simulink model "fft_test"  (Simulink 7.0)
settings: Solver=VariableStepDiscrete  StartTime=0.0  StopTime=500  RelTol=1e-3
undefined symbols (not defined in the file or in its folder): bit_rev
libraries: xbsIndex_r4 x960, casper_library x89
(part 1 of 10)
settings Model: Creator=User  LastModifiedBy=User
settings DebuggingCC: SaveWithDisabledLinksMsg=none  SaveWithParameterizedLinksMsg=none

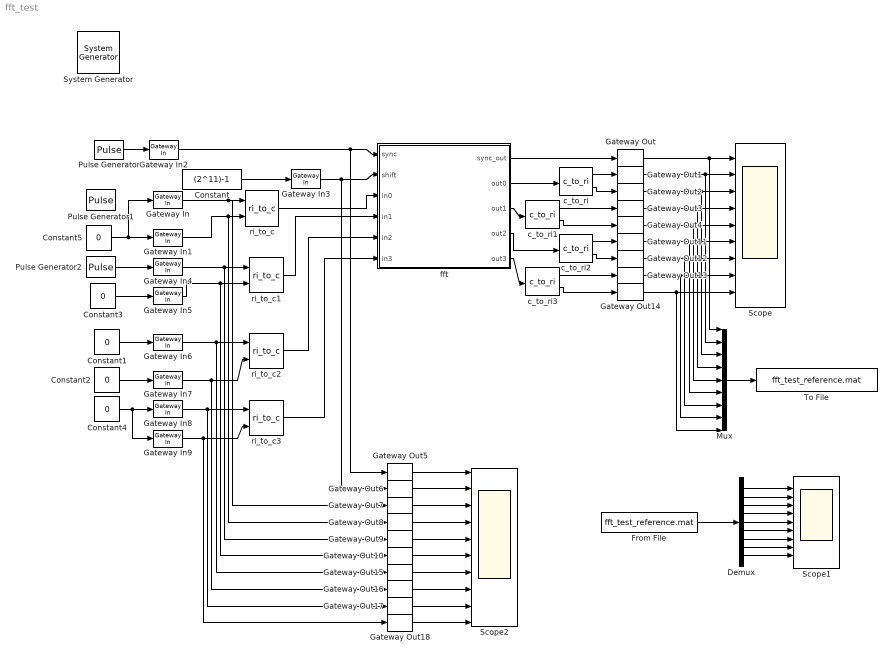
== system fft_test ==
  " System Generator" : xbsIndex_r4/ System Generator  Tag=genX  SystemSampleTime=-1  xilinxfamily=Virtex4  part=xc4vsx35  speed=-10  package=ff668  synthesis_tool=XST  clock_wrapper=Clock Enables  directory=./netlist  testbench=off  simulink_period=1  sysclk_period=100  dcm_input_clock_period=100  incr_netlist=off  trim_vbits=Everywhere in SubSystem  dbl_ovrd=According to Block Masks  core_generation=According to Block Masks  run_coregen=off  deprecated_control=off  eval_field=0  block_type=sysgen
      settings: block_version=10.1.1
  Constant : Constant  Value=(2^11)-1  OutDataType=sfix(16)  OutScaling=2^0
  Constant{1..5} (5 alike) : Constant  Value=0  OutDataType=sfix(16)  OutScaling=2^0
  Demux : Demux  Outputs=9
  From File : FromFile  FileName=fft_test_reference.mat  SampleTime=1
  Gateway In{,1,4..9} (8 alike) : xbsIndex_r4/Gateway In  arith_type="Signed  (2's comp)"  n_bits=8  bin_pt=7  quantization=Truncate  overflow=Wrap  period=1  dbl_ovrd=off  timing_constraint=None  locs_specified=off  LOCs={}  block_type=gatewayin
      settings: infoedit="Gateway in block.  Converts inputs of type Simulink integer, double and fixed point to  Xilinx fixed point type.<P><P>Hardware notes:  In hardware these blocks become top level input ports."  block_version=10.1.1
  Gateway In2 : xbsIndex_r4/Gateway In  arith_type=Boolean  n_bits=18  bin_pt=17  quantization=Truncate  overflow=Wrap  period=1  dbl_ovrd=off  timing_constraint=None  locs_specified=off  LOCs={}  block_type=gatewayin
      settings: infoedit="Gateway in block.  Converts inputs of type Simulink integer, double and fixed point to  Xilinx fixed point type.<P><P>Hardware notes:  In hardware these blocks become top level input ports."  block_version=10.1.1
  Gateway In3 : xbsIndex_r4/Gateway In  arith_type=Unsigned  n_bits=11  bin_pt=0  quantization=Truncate  overflow=Wrap  period=1  dbl_ovrd=off  timing_constraint=None  locs_specified=off  LOCs={}  block_type=gatewayin
      settings: infoedit="Gateway in block.  Converts inputs of type Simulink integer, double and fixed point to  Xilinx fixed point type.<P><P>Hardware notes:  In hardware these blocks become top level input ports."  block_version=10.1.1
  Gateway Out{,1..18} (19 alike) : xbsIndex_r4/Gateway Out  hdl_port=on  timing_constraint=None  locs_specified=off  LOCs={}  block_type=gatewayout
      settings: infoedit="Gateway out block.  Converts Xilinx fixed point inputs into ouputs of type Simulink integer, double, or fixed point.<P><P>Hardware notes:  In hardware these blocks become top level output ports or are discarded, depending on how they are configured."  block_version=10.1.1
  Mux : Mux  Inputs=9
  Pulse Generator : DiscretePulseGenerator  Period=2^7  PhaseDelay=11
  Pulse Generator1 : DiscretePulseGenerator  Amplitude=0.5  Period=2^4  PhaseDelay=12
  Pulse Generator2 : DiscretePulseGenerator  Amplitude=0.5  Period=2^5  PhaseDelay=12
  Scope : Scope  NumInputPorts=9
      settings: YMin=-1~0~0~-5~-5~-5~-5~-5~-5  YMax=2~1~1~5~5~5~5~5~5
  Scope1 : Scope  NumInputPorts=9
      settings: YMin=-1~0~0~-5~-5~-5~-5~-5~-5  YMax=2~1~1~5~5~5~5~5~5
  Scope2 : Scope  NumInputPorts=10
      settings: YMin=-1~0~0~-5~-5~-5~-5~-5~-5~-5  YMax=2~1~1~5~5~5~5~5~5~5  SaveName=ScopeData2
  To File : ToFile  Filename=fft_test_reference.mat  MatrixName=reference
  c_to_ri{,1..3} (4 alike) : casper_library/Misc/c_to_ri  SystemSampleTime=-1  n_bits=8  bin_pt=7
      settings: AttributesFormatString=8_7 r/i
  fft : Subsystem  AncestorBlock=casper_library/FFTs/fft  mask(fft){FFTSize=6, BitWidth=8, n_inputs=2, quantization=Round  (unbiased: +/- Inf), overflow=Saturate, add_latency=2, mult_latency=3, bram_latency=1}
      mask prompts: FFTSize "Size of FFT: (2^?)"; BitWidth "Bit Width"; n_inputs "Number of Simultaneous Inputs: (2^?)"; quantization "Quantization Behavior"; overflow "Overflow Behavior"; add_latency "Add Latency"; mult_latency "Mult Latency"; bram_latency "BRAM Latency"
      mask init:
      | fft_init(gcb,...
      |     'FFTSize', FFTSize,...
      |     'BitWidth', BitWidth,...
      |     'n_inputs', n_inputs,...
      |     'quantization', quantization,...
      |     'overflow', overflow,...
      |     'add_latency', add_latency,...
      |     'mult_latency', mult_latency,...
      |     'bram_latency', bram_latency);
      settings: AttributesFormatString=FFTSize=6, n_inputs=2
      mask StyleString: edit,edit,edit,popup(Truncate|Round  (unbiased: +/- Inf)|Round  (unbiased: Even Values)),popup(Wrap|Saturate|Error),edit,edit,edit
  ri_to_c{,1..3} (4 alike) : casper_library/Misc/ri_to_c  SystemSampleTime=-1
  wires:
  Pulse Generator/1 -> Gateway In2/1
  Gateway In2/1 -> fft/1(sync), Gateway Out5/1
  Constant/1 -> Gateway In3/1
  Gateway In3/1 -> fft/2(shift), Gateway Out6/1
  fft/1(sync_out) -> Gateway Out/1
  fft/2(out0) -> c_to_ri/1
  c_to_ri/1 -> Gateway Out1/1
  c_to_ri/2 -> Gateway Out2/1
  c_to_ri1/2 -> Gateway Out4/1
  fft/3(out1) -> c_to_ri1/1
  c_to_ri1/1 -> Gateway Out3/1
  Gateway Out/1 -> Scope/1, Mux/1
  Gateway In/1 -> ri_to_c/1, Gateway Out7/1
  Gateway In1/1 -> ri_to_c/2, Gateway Out8/1
  Gateway In4/1 -> ri_to_c1/1, Gateway Out9/1
  Gateway In5/1 -> ri_to_c1/2, Gateway Out10/1
  Gateway Out1/1 -> Scope/2, Mux/2
  Gateway Out2/1 -> Scope/3, Mux/3
  Mux/1 -> To File/1
  Demux/1 -> Scope1/1
  Demux/2 -> Scope1/2
  Demux/3 -> Scope1/3
  Demux/4 -> Scope1/4
  Demux/5 -> Scope1/5
  Gateway Out5/1 -> Scope2/1
  Gateway Out6/1 -> Scope2/2
  Gateway Out7/1 -> Scope2/3
  Gateway Out8/1 -> Scope2/4
  Gateway Out9/1 -> Scope2/5
  Gateway Out10/1 -> Scope2/6
  Constant2/1 -> Gateway In7/1
  Constant4/1 -> Gateway In8/1, Gateway In9/1
  Gateway In6/1 -> ri_to_c2/1, Gateway Out15/1
  Gateway In7/1 -> ri_to_c2/2, Gateway Out16/1
  Gateway In8/1 -> ri_to_c3/1, Gateway Out17/1
  Gateway In9/1 -> ri_to_c3/2, Gateway Out18/1
  ri_to_c/1 -> fft/3(in0)
  ri_to_c1/1 -> fft/4(in1)
  ri_to_c2/1 -> fft/5(in2)
  ri_to_c3/1 -> fft/6(in3)
  fft/4(out2) -> c_to_ri2/1
  fft/5(out3) -> c_to_ri3/1
  c_to_ri2/1 -> Gateway Out11/1
  c_to_ri2/2 -> Gateway Out12/1
  c_to_ri3/1 -> Gateway Out13/1
  c_to_ri3/2 -> Gateway Out14/1
  Gateway Out3/1 -> Scope/4, Mux/4
  Gateway Out4/1 -> Scope/5, Mux/5
  Gateway Out11/1 -> Scope/6, Mux/6
  Gateway Out12/1 -> Scope/7, Mux/7
  Gateway Out13/1 -> Scope/8, Mux/8
  Gateway Out14/1 -> Scope/9, Mux/9
  Gateway Out15/1 -> Scope2/7
  Gateway Out16/1 -> Scope2/8
  Gateway Out17/1 -> Scope2/9
  Gateway Out18/1 -> Scope2/10
  From File/1 -> Demux/1
  Demux/6 -> Scope1/6
  Demux/7 -> Scope1/7
  Demux/8 -> Scope1/8
  Demux/9 -> Scope1/9
  Constant3/1 -> Gateway In5/1
  Constant1/1 -> Gateway In6/1
  Pulse Generator2/1 -> Gateway In4/1
  Constant5/1 -> Gateway In1/1, Gateway In/1

== system fft_test/fft ==
  sync : Inport  OutDataType=sfix(16)  OutScaling=2^0
  shift : Inport  Port=2  OutDataType=sfix(16)  OutScaling=2^0
  in0 : Inport  Port=3
  in1 : Inport  Port=4
  in2 : Inport  Port=5
  in3 : Inport  Port=6
  fft_biplex0 : Subsystem  AncestorBlock=casper_library/FFTs/fft_biplex  mask(fft_biplex){FFTSize=4, BitWidth=8, quantization=Round  (unbiased: +/- Inf), overflow=Saturate, add_latency=2, mult_latency=3, bram_latency=1}
      mask prompts: FFTSize "Size of FFT: (2^? pnts)"; BitWidth "Bitwidth: (Max Efficiency at 18 bits)"; quantization "Quantization Behavior"; overflow "Overflow Behavior"; add_latency "Add Latency"; mult_latency "Mult Latency"; bram_latency "BRAM Latency"
      mask init:
      | fft_biplex_init(gcb,...
      |     'FFTSize', FFTSize,...
      |     'BitWidth', BitWidth,...
      |     'quantization', quantization,...
      |     'overflow', overflow,...
      |     'add_latency', add_latency,...
      |     'mult_latency', mult_latency,...
      |     'bram_latency', bram_latency);
      settings: AttributesFormatString=FFTSize=4, BitWidth=8
      mask StyleString: edit,edit,popup(Truncate|Round  (unbiased: +/- Inf)|Round  (unbiased: Even Values)),popup(Wrap|Saturate|Error),edit,edit,edit
  fft_biplex1 : Subsystem  AncestorBlock=casper_library/FFTs/fft_biplex  mask(fft_biplex){FFTSize=4, BitWidth=8, quantization=Round  (unbiased: +/- Inf), overflow=Saturate, add_latency=2, mult_latency=3, bram_latency=1}
      mask prompts: FFTSize "Size of FFT: (2^? pnts)"; BitWidth "Bitwidth: (Max Efficiency at 18 bits)"; quantization "Quantization Behavior"; overflow "Overflow Behavior"; add_latency "Add Latency"; mult_latency "Mult Latency"; bram_latency "BRAM Latency"
      mask init: same as fft_test/fft/fft_biplex0
      settings: AttributesFormatString=FFTSize=4, BitWidth=8
      mask StyleString: edit,edit,popup(Truncate|Round  (unbiased: +/- Inf)|Round  (unbiased: Even Values)),popup(Wrap|Saturate|Error),edit,edit,edit
  fft_direct : Subsystem  AncestorBlock=casper_library/FFTs/fft_direct  mask(fft_direct){FFTSize=2, BitWidth=8, add_latency=2, mult_latency=3, bram_latency=1, quantization=Round  (unbiased: +/- Inf), overflow=Saturate, MapTail=1, LargerFFTSize=6, StartStage=5}
      mask prompts: FFTSize "Size of FFT: (2^?)"; BitWidth "Bit Width"; add_latency "Add Latency"; mult_latency "Mult Latency"; bram_latency "BRAM Latency"; quantization "Quantization Behavior"; overflow "Overflow Behavior"; MapTail "Map Tail of Larger FFT"; LargerFFTSize "Size of Larger FFT (2^?):"; StartStage "Start Stage of Map Tail:"
      mask help:
      | Implements an N-point FFT with the classic
      | butterfly structure with N inputs and N outputs
      mask init:
      | fft_direct_init(gcb,...
      |     'FFTSize', FFTSize,...
      |     'BitWidth', BitWidth,...
      |     'add_latency', add_latency,...
      |     'mult_latency', mult_latency,...
      |     'bram_latency', bram_latency,...
      |     'quantization', quantization,...
      |     'overflow', overflow,...
      |     'MapTail', MapTail,...
      |     'LargerFFTSize', LargerFFTSize,...
      |     'StartStage', StartStage);
      settings: AttributesFormatString=FFTSize=2
      mask StyleString: edit,edit,edit,edit,edit,popup(Truncate|Round  (unbiased: +/- Inf)|Round  (unbiased: Even Values)),popup(Wrap|Saturate|Error),edit,edit,edit
  fft_unscrambler : Subsystem  AncestorBlock=casper_library/FFTs/fft_unscrambler  mask(fft_unscrambler){FFTSize=6, n_inputs=2, bram_latency=1}
      mask prompts: FFTSize "Size of FFT: (2^?)"; n_inputs "Number of Simultaneous Inputs: (2^?)"; bram_latency "BRAM Latency"
      mask init:
      | fft_unscrambler_init(gcb,...
      |     'FFTSize',FFTSize,... 
      |     'n_inputs', n_inputs,...
      |     'bram_latency', bram_latency);
      settings: AttributesFormatString=FFTSize=6, n_inputs=2
  slice : xbsIndex_r4/Slice  nbits=2  boolean_output=off  mode=Lower Bit Location + Width  bit1=0  base1=MSB of Input  bit0=4  base0=LSB of Input  dbl_ovrd=off  block_type=slice
      settings: infoedit="Extracts a given range of bits from each input sample and presents it at the output.  The output type is ordinarily unsigned with binary point at zero, but can be Boolean when the slice is one bit wide.<P><P>Hardware notes: In hardware this block costs nothing."  block_version=10.1.1
  sync_out : Outport  OutDataType=sfix(16)  OutScaling=2^0
  out0 : Outport  Port=2  OutDataType=sfix(16)  OutScaling=2^0
  out1 : Outport  Port=3  OutDataType=sfix(16)  OutScaling=2^0
  out2 : Outport  Port=4
  out3 : Outport  Port=5
  wires:
  in0/1 -> fft_biplex0/1(pol1)
  in1/1 -> fft_biplex0/2(pol2)
  shift/1 -> fft_biplex0/4(shift), fft_biplex1/4(shift), slice/1
  sync/1 -> fft_biplex0/3(sync), fft_biplex1/3(sync)
  in2/1 -> fft_biplex1/1(pol1)
  in3/1 -> fft_biplex1/2(pol2)
  slice/1 -> fft_direct/2(shift)
  fft_biplex0/4(sync_out) -> fft_direct/1(sync)
  fft_biplex0/1(pol1_out) -> fft_direct/3(in0)
  fft_biplex0/2(pol2_out) -> fft_direct/4(in1)
  fft_biplex1/1(pol1_out) -> fft_direct/5(in2)
  fft_biplex1/2(pol2_out) -> fft_direct/6(in3)
  fft_direct/1(sync_out) -> fft_unscrambler/1(sync)
  fft_unscrambler/1(sync_out) -> sync_out/1
  fft_direct/2(out0) -> fft_unscrambler/2(In1)
  fft_unscrambler/2(Out1) -> out0/1
  fft_direct/3(out1) -> fft_unscrambler/3(In2)
  fft_unscrambler/3(Out2) -> out1/1
  fft_direct/4(out2) -> fft_unscrambler/4(In3)
  fft_unscrambler/4(Out3) -> out2/1
  fft_direct/5(out3) -> fft_unscrambler/5(In4)
  fft_unscrambler/5(Out4) -> out3/1

== system fft_test/fft/fft_biplex0 ==
  pol1 : Inport  OutDataType=sfix(16)  OutScaling=2^0
  pol2 : Inport  Port=2  OutDataType=sfix(16)  OutScaling=2^0
  sync : Inport  Port=3  OutDataType=sfix(16)  OutScaling=2^0
  shift : Inport  Port=4  OutDataType=sfix(16)  OutScaling=2^0
  biplex_core : Subsystem  AncestorBlock=casper_library/FFTs/biplex_core  mask(biplex_core){FFTSize=4, BitWidth=8, quantization=Round  (unbiased: +/- Inf), overflow=Saturate, add_latency=2, mult_latency=3, bram_latency=1}
      mask prompts: FFTSize "Size of FFT: (2^? pnts)"; BitWidth "Bitwidth: (Max Efficiency at 18 bits)"; quantization "Quantization Behavior"; overflow "Overflow Behavior"; add_latency "Add Latency"; mult_latency "Mult Latency"; bram_latency "BRAM Latency"
      mask init:
      | biplex_core_init(gcb,...
      |     'FFTSize', FFTSize,...
      |     'BitWidth', BitWidth,...
      |     'quantization', quantization,...
      |     'overflow', overflow,...
      |     'add_latency', add_latency,...
      |     'mult_latency', mult_latency,...
      |     'bram_latency', bram_latency);
      settings: AttributesFormatString=FFTSize=4
      mask StyleString: edit,edit,popup(Truncate|Round  (unbiased: +/- Inf)|Round  (unbiased: Even Values)),popup(Wrap|Saturate|Error),edit,edit,edit
  biplex_cplx_unscrambler : Subsystem  mask{FFTSize=4, bram_latency=1}
      mask prompts: FFTSize "Size of FFT: (2^? pnts)"; bram_latency "BRAM Latency"
      mask init:
      | blk = gcb;
      | map = bit_reverse(0:2^(FFTSize-1)-1, FFTSize-1);
      | set_param([blk,'/reorder'],'map',mat2str([map,map+2^(FFTSize-1)]));
      | set_param([blk,'/reorder'],'bram_latency', num2str(bram_latency));
      | set_param([blk,'/reorder1'],'map',mat2str([map+2^(FFTSize-1),map]));
      | set_param([blk,'/reorder1'],'bram_latency', num2str(bram_latency));
  pol1_out : Outport  OutDataType=sfix(16)  OutScaling=2^0
  pol2_out : Outport  Port=2  OutDataType=sfix(16)  OutScaling=2^0
  of : Outport  Port=3  OutDataType=sfix(16)  OutScaling=2^0
  sync_out : Outport  Port=4  OutDataType=sfix(16)  OutScaling=2^0
  wires:
  biplex_cplx_unscrambler/3(sync_out) -> sync_out/1
  biplex_cplx_unscrambler/2(pol2) -> pol2_out/1
  biplex_core/4(sync_out) -> biplex_cplx_unscrambler/3(sync)
  biplex_core/2(out2) -> biplex_cplx_unscrambler/2(odd)
  biplex_core/1(out1) -> biplex_cplx_unscrambler/1(even)
  pol1/1 -> biplex_core/1(pol1)
  pol2/1 -> biplex_core/2(pol2)
  sync/1 -> biplex_core/3(sync)
  shift/1 -> biplex_core/4(shift)
  biplex_cplx_unscrambler/1(pol1) -> pol1_out/1
  biplex_core/3(of) -> of/1

== system fft_test/fft/fft_biplex1 ==
  pol1 : Inport  OutDataType=sfix(16)  OutScaling=2^0
  pol2 : Inport  Port=2  OutDataType=sfix(16)  OutScaling=2^0
  sync : Inport  Port=3  OutDataType=sfix(16)  OutScaling=2^0
  shift : Inport  Port=4  OutDataType=sfix(16)  OutScaling=2^0
  biplex_core : Subsystem  AncestorBlock=casper_library/FFTs/biplex_core  mask(biplex_core){FFTSize=4, BitWidth=8, quantization=Round  (unbiased: +/- Inf), overflow=Saturate, add_latency=2, mult_latency=3, bram_latency=1}
      mask prompts: FFTSize "Size of FFT: (2^? pnts)"; BitWidth "Bitwidth: (Max Efficiency at 18 bits)"; quantization "Quantization Behavior"; overflow "Overflow Behavior"; add_latency "Add Latency"; mult_latency "Mult Latency"; bram_latency "BRAM Latency"
      mask init: same as fft_test/fft/fft_biplex0/biplex_core
      settings: AttributesFormatString=FFTSize=4
      mask StyleString: edit,edit,popup(Truncate|Round  (unbiased: +/- Inf)|Round  (unbiased: Even Values)),popup(Wrap|Saturate|Error),edit,edit,edit
  biplex_cplx_unscrambler : Subsystem  mask{FFTSize=4, bram_latency=1}
      mask prompts: FFTSize "Size of FFT: (2^? pnts)"; bram_latency "BRAM Latency"
      mask init: same as fft_test/fft/fft_biplex0/biplex_cplx_unscrambler
  pol1_out : Outport  OutDataType=sfix(16)  OutScaling=2^0
  pol2_out : Outport  Port=2  OutDataType=sfix(16)  OutScaling=2^0
  of : Outport  Port=3  OutDataType=sfix(16)  OutScaling=2^0
  sync_out : Outport  Port=4  OutDataType=sfix(16)  OutScaling=2^0
  wires:
  biplex_cplx_unscrambler/3(sync_out) -> sync_out/1
  biplex_cplx_unscrambler/2(pol2) -> pol2_out/1
  biplex_core/4(sync_out) -> biplex_cplx_unscrambler/3(sync)
  biplex_core/2(out2) -> biplex_cplx_unscrambler/2(odd)
  biplex_core/1(out1) -> biplex_cplx_unscrambler/1(even)
  pol1/1 -> biplex_core/1(pol1)
  pol2/1 -> biplex_core/2(pol2)
  sync/1 -> biplex_core/3(sync)
  shift/1 -> biplex_core/4(shift)
  biplex_cplx_unscrambler/1(pol1) -> pol1_out/1
  biplex_core/3(of) -> of/1

== system fft_test/fft/fft_direct ==
  sync : Inport  OutDataType=sfix(16)  OutScaling=2^0
  shift : Inport  Port=2  OutDataType=sfix(16)  OutScaling=2^0
  in0 : Inport  Port=3  OutDataType=sfix(16)  OutScaling=2^0
  in1 : Inport  Port=4  OutDataType=sfix(16)  OutScaling=2^0
  in2 : Inport  Port=5  OutDataType=sfix(16)  OutScaling=2^0
  in3 : Inport  Port=6  OutDataType=sfix(16)  OutScaling=2^0
  butterfly1_0 : Subsystem  AncestorBlock=casper_library/FFTs/butterfly_direct  mask(butterfly_direct){FFTSize=6, Coeffs=[0 8 4 12 2 10 6 14 1 9 5 13 3 11 7 15], StepPeriod=0, BitWidth=8, add_latency=2, mult_latency=3, bram_latency=1, use_bram=1, quantization=Round  (unbiased: +/- Inf), overflow=Saturate}
      mask prompts: FFTSize "Size of FFT: (2^?)"; Coeffs "Coefficients: (0 to 2^(FFTSize-1)-1)"; StepPeriod "Coefficient Step Period: (2^?)"; BitWidth "Output Bitwidth:"; add_latency "Add Latency"; mult_latency "Mult Latency"; bram_latency "BRAM Latency"; use_bram "Store Coefficients in BRAM"; quantization "Quantization Behavior"; overflow "Overflow Behavior"
      mask init:
      | butterfly_direct_init(gcb,...
      |               'FFTSize', FFTSize,...
      |               'Coeffs', Coeffs,...
      |               'StepPeriod', StepPeriod,...
      |               'BitWidth', BitWidth,...
      |               'add_latency', add_latency,...
      |               'mult_latency', mult_latency,...
      |               'bram_latency', bram_latency,...
      |               'use_bram',use_bram,...
      |               'quantization',quantization,...
      |               'overflow',overflow);
      settings: AttributesFormatString=|
      | FFTSize=6, Coeffs=[0   8   4  12   2  10   6  14   1   9   5  13   3  11   7  15],
      |  StepPeriod=0, BitWidth=8
      mask StyleString: edit,edit,edit,edit,edit,edit,edit,edit,popup(Truncate|Round  (unbiased: +/- Inf)|Round  (unbiased: Even Values)),popup(Wrap|Saturate|Error)
  butterfly1_1 : Subsystem  AncestorBlock=casper_library/FFTs/butterfly_direct  mask(butterfly_direct){FFTSize=6, Coeffs=[0 8 4 12 2 10 6 14 1 9 5 13 3 11 7 15], StepPeriod=0, BitWidth=8, add_latency=2, mult_latency=3, bram_latency=1, use_bram=1, quantization=Round  (unbiased: +/- Inf), overflow=Saturate}
      mask prompts: FFTSize "Size of FFT: (2^?)"; Coeffs "Coefficients: (0 to 2^(FFTSize-1)-1)"; StepPeriod "Coefficient Step Period: (2^?)"; BitWidth "Output Bitwidth:"; add_latency "Add Latency"; mult_latency "Mult Latency"; bram_latency "BRAM Latency"; use_bram "Store Coefficients in BRAM"; quantization "Quantization Behavior"; overflow "Overflow Behavior"
      mask init: same as fft_test/fft/fft_direct/butterfly1_0
      settings: AttributesFormatString=|
      | FFTSize=6, Coeffs=[0   8   4  12   2  10   6  14   1   9   5  13   3  11   7  15],
      |  StepPeriod=0, BitWidth=8
      mask StyleString: edit,edit,edit,edit,edit,edit,edit,edit,popup(Truncate|Round  (unbiased: +/- Inf)|Round  (unbiased: Even Values)),popup(Wrap|Saturate|Error)
  butterfly2_0 : Subsystem  AncestorBlock=casper_library/FFTs/butterfly_direct  mask(butterfly_direct){FFTSize=6, Coeffs=[0 16 8 24 4 20 12 28 2 18 10 26 6 22 14 30], StepPeriod=0, BitWidth=8, add_latency=2, mult_latency=3, bram_latency=1, use_bram=1, quantization=Round  (unbiased: +/- Inf), overflow=Saturate}
      mask prompts: FFTSize "Size of FFT: (2^?)"; Coeffs "Coefficients: (0 to 2^(FFTSize-1)-1)"; StepPeriod "Coefficient Step Period: (2^?)"; BitWidth "Output Bitwidth:"; add_latency "Add Latency"; mult_latency "Mult Latency"; bram_latency "BRAM Latency"; use_bram "Store Coefficients in BRAM"; quantization "Quantization Behavior"; overflow "Overflow Behavior"
      mask init: same as fft_test/fft/fft_direct/butterfly1_0
      settings: AttributesFormatString=|
      | FFTSize=6, Coeffs=[0  16   8  24   4  20  12  28   2  18  10  26   6  22  14  30],
      |  StepPeriod=0, BitWidth=8
      mask StyleString: edit,edit,edit,edit,edit,edit,edit,edit,popup(Truncate|Round  (unbiased: +/- Inf)|Round  (unbiased: Even Values)),popup(Wrap|Saturate|Error)
  butterfly2_1 : Subsystem  AncestorBlock=casper_library/FFTs/butterfly_direct  mask(butterfly_direct){FFTSize=6, Coeffs=[1 17 9 25 5 21 13 29 3 19 11 27 7 23 15 31], StepPeriod=0, BitWidth=8, add_latency=2, mult_latency=3, bram_latency=1, use_bram=1, quantization=Round  (unbiased: +/- Inf), overflow=Saturate}
      mask prompts: FFTSize "Size of FFT: (2^?)"; Coeffs "Coefficients: (0 to 2^(FFTSize-1)-1)"; StepPeriod "Coefficient Step Period: (2^?)"; BitWidth "Output Bitwidth:"; add_latency "Add Latency"; mult_latency "Mult Latency"; bram_latency "BRAM Latency"; use_bram "Store Coefficients in BRAM"; quantization "Quantization Behavior"; overflow "Overflow Behavior"
      mask init: same as fft_test/fft/fft_direct/butterfly1_0
      settings: AttributesFormatString=|
      | FFTSize=6, Coeffs=[1  17   9  25   5  21  13  29   3  19  11  27   7  23  15  31],
      |  StepPeriod=0, BitWidth=8
      mask StyleString: edit,edit,edit,edit,edit,edit,edit,edit,popup(Truncate|Round  (unbiased: +/- Inf)|Round  (unbiased: Even Values)),popup(Wrap|Saturate|Error)
  node0_{0..3} (4 alike) : xbsIndex_r4/Delay  en=off  latency=0  dbl_ovrd=off  reg_retiming=off  block_type=delay
      settings: xl_area=[0, 0, 0, 0, 0, 0, 0]  block_version=9.1.01
  node1_{0..3} (4 alike) : xbsIndex_r4/Delay  en=off  latency=0  dbl_ovrd=off  reg_retiming=off  block_type=delay
      settings: xl_area=[0, 0, 0, 0, 0, 0, 0]  block_version=9.1.01
  node2_{0..3} (4 alike) : xbsIndex_r4/Delay  en=off  latency=0  dbl_ovrd=off  reg_retiming=off  block_type=delay
      settings: xl_area=[0, 0, 0, 0, 0, 0, 0]  block_version=9.1.01
  slice0 : xbsIndex_r4/Slice  nbits=1  boolean_output=on  mode=Lower Bit Location + Width  bit1=0  base1=MSB of Input  bit0=0  base0=LSB of Input  dbl_ovrd=off  block_type=slice
      settings: infoedit="Extracts a given range of bits from each input sample and presents it at the output.  The output type is ordinarily unsigned with binary point at zero, but can be Boolean when the slice is one bit wide.<P><P>Hardware notes: In hardware this block costs nothing."  block_version=9.1.01
  slice1 : xbsIndex_r4/Slice  nbits=1  boolean_output=on  mode=Lower Bit Location + Width  bit1=0  base1=MSB of Input  bit0=1  base0=LSB of Input  dbl_ovrd=off  block_type=slice
      settings: infoedit="Extracts a given range of bits from each input sample and presents it at the output.  The output type is ordinarily unsigned with binary point at zero, but can be Boolean when the slice is one bit wide.<P><P>Hardware notes: In hardware this block costs nothing."  block_version=9.1.01
  sync_out : Outport  OutDataType=sfix(16)  OutScaling=2^0
  out0 : Outport  Port=2  OutDataType=sfix(16)  OutScaling=2^0
  out1 : Outport  Port=3  OutDataType=sfix(16)  OutScaling=2^0
  out2 : Outport  Port=4  OutDataType=sfix(16)  OutScaling=2^0
  out3 : Outport  Port=5  OutDataType=sfix(16)  OutScaling=2^0
  wires:
  in0/1 -> node0_0/1
  in1/1 -> node0_1/1
  in2/1 -> node0_2/1
  in3/1 -> node0_3/1
  shift/1 -> slice0/1, slice1/1
  node2_0/1 -> out0/1
  node2_1/1 -> out2/1
  node2_2/1 -> out1/1
  node2_3/1 -> out3/1
  node0_0/1 -> butterfly1_0/1(a)
  node0_2/1 -> butterfly1_0/2(b)
  butterfly1_0/1(a+bw) -> node1_0/1
  butterfly1_0/2(a-bw) -> node1_2/1
  sync/1 -> butterfly1_0/3(sync), butterfly1_1/3(sync)
  slice0/1 -> butterfly1_0/4(shift), butterfly1_1/4(shift)
  node0_1/1 -> butterfly1_1/1(a)
  node0_3/1 -> butterfly1_1/2(b)
  butterfly1_1/1(a+bw) -> node1_1/1
  butterfly1_1/2(a-bw) -> node1_3/1
  node1_0/1 -> butterfly2_0/1(a)
  node1_1/1 -> butterfly2_0/2(b)
  butterfly2_0/1(a+bw) -> node2_0/1
  butterfly2_0/2(a-bw) -> node2_1/1
  butterfly1_0/4(sync_out) -> butterfly2_0/3(sync)
  butterfly2_0/4(sync_out) -> sync_out/1
  slice1/1 -> butterfly2_0/4(shift), butterfly2_1/4(shift)
  node1_2/1 -> butterfly2_1/1(a)
  node1_3/1 -> butterfly2_1/2(b)
  butterfly2_1/1(a+bw) -> node2_2/1
  butterfly2_1/2(a-bw) -> node2_3/1
  butterfly1_1/4(sync_out) -> butterfly2_1/3(sync)

== system fft_test/fft/fft_unscrambler ==
  sync : Inport  OutDataType=sfix(16)  OutScaling=2^0
  In1 : Inport  Port=2  OutDataType=sfix(16)  OutScaling=2^0
  In2 : Inport  Port=3  OutDataType=sfix(16)  OutScaling=2^0
  In3 : Inport  Port=4
  In4 : Inport  Port=5
  const : xbsIndex_r4/Constant  arith_type=Boolean  const=1  n_bits=1  bin_pt=0  explicit_period=on  period=1  equ=P=C  opselect=C  inp2=PCIN>>17  opr=+  inp1=P  carry=CIN  dbl_ovrd=off  block_type=constant
      settings: block_version=9.1.01
  reorder : Subsystem  AncestorBlock=casper_library/Reorder/reorder  mask(reorder){map=[0 4 8 12 1 5 9 13 2 6 10 14 3 7 11 15], n_inputs=4, bram_latency=1, map_latency=1, double_buffer=0}
      mask prompts: map "Output Order:"; n_inputs "Number of inputs"; bram_latency "BRAM Latency"; map_latency "Map Latency"; double_buffer "Double Buffer"
      mask init:
      | reorder_init(gcb, ...
      |     'map', map, ...
      |     'n_inputs', n_inputs, ...
      |     'bram_latency', bram_latency, ...
      |     'map_latency', map_latency, ...
      |     'double_buffer', double_buffer);
      settings: AttributesFormatString=order=2
  square_transposer : Subsystem  AncestorBlock=casper_library/Reorder/square_transposer  mask(square_transposer){n_inputs=2}
      mask prompts: n_inputs "Number of inputs (2^?):"
      mask init:
      | square_transposer_init(gcb,...
      |     'n_inputs', n_inputs);
      settings: AttributesFormatString=n_inputs=2
  sync_out : Outport  OutDataType=sfix(16)  OutScaling=2^0
  Out1 : Outport  Port=2  OutDataType=sfix(16)  OutScaling=2^0
  Out2 : Outport  Port=3  OutDataType=sfix(16)  OutScaling=2^0
  Out3 : Outport  Port=4
  Out4 : Outport  Port=5
  wires:
  sync/1 -> square_transposer/1(sync)
  square_transposer/1(sync_out) -> reorder/1(sync)
  reorder/1(sync_out) -> sync_out/1
  const/1 -> reorder/2(en)
  In1/1 -> square_transposer/2(In1)
  square_transposer/2(Out1) -> reorder/3(din0)
  reorder/3(dout0) -> Out1/1
  In2/1 -> square_transposer/3(In2)
  square_transposer/3(Out2) -> reorder/4(din1)
  reorder/4(dout1) -> Out2/1
  In3/1 -> square_transposer/4(In3)
  square_transposer/4(Out3) -> reorder/5(din2)
  reorder/5(dout2) -> Out3/1
  In4/1 -> square_transposer/5(In4)
  square_transposer/5(Out4) -> reorder/6(din3)
  reorder/6(dout3) -> Out4/1

== system fft_test/fft/fft_biplex0/biplex_core ==
  pol1 : Inport  OutDataType=sfix(16)  OutScaling=2^0
  pol2 : Inport  Port=2  OutDataType=sfix(16)  OutScaling=2^0
  sync : Inport  Port=3  OutDataType=sfix(16)  OutScaling=2^0
  shift : Inport  Port=4  OutDataType=sfix(16)  OutScaling=2^0
  fft_stage_1 : Subsystem  mask(fft_stage_n){FFTSize=4, FFTStage=1, BitWidth=8, use_bram=0, CoeffBram=0, MaxCoeffNum=11, quantization=Round  (unbiased: +/- Inf), overflow=Saturate, add_latency=2, mult_latency=3, bram_latency=1}
      mask prompts: FFTSize "Size of FFT: (2^? pnts)"; FFTStage "Stage of FFT:"; BitWidth "Output Bitwidth:"; use_bram "Implement Delays in BRAM:"; CoeffBram "Store Coefficients in BRAM:"; MaxCoeffNum "Maximum Coefficient Depth: (2^?)"; quantization "Quantization Behavior"; overflow "Overflow Behavior"; add_latency "Add Latency"; mult_latency "Mult Latency"; bram_latency "BRAM Latency"
      mask init:
      | fft_stage_n_init(gcb,...
      |     'FFTSize', FFTSize,...
      |     'FFTStage', FFTStage,...
      |     'BitWidth', BitWidth,...
      |     'use_bram', use_bram,...
      |     'CoeffBram', CoeffBram,...
      |     'MaxCoeffNum', MaxCoeffNum,...
      |     'quantization', quantization,...
      |     'overflow', overflow,...
      |     'add_latency', add_latency,...
      |     'mult_latency', mult_latency,...
      |     'bram_latency', bram_latency);
      settings: AttributesFormatString=FFTSize=4, FFTStage=1, BitWidth=8
      mask StyleString: edit,edit,edit,edit,edit,edit,popup(Truncate|Round  (unbiased: +/- Inf)|Round  (unbiased: Even Values)),popup(Wrap|Saturate|Error),edit,edit,edit
  fft_stage_2 : Subsystem  AncestorBlock=casper_library/FFTs/fft_stage_n  mask(fft_stage_n){FFTSize=4, FFTStage=2, BitWidth=8, use_bram=0, CoeffBram=0, MaxCoeffNum=11, quantization=Round  (unbiased: +/- Inf), overflow=Saturate, add_latency=2, mult_latency=3, bram_latency=1}
      mask prompts: FFTSize "Size of FFT: (2^? pnts)"; FFTStage "Stage of FFT:"; BitWidth "Output Bitwidth:"; use_bram "Implement Delays in BRAM:"; CoeffBram "Store Coefficients in BRAM:"; MaxCoeffNum "Maximum Coefficient Depth: (2^?)"; quantization "Quantization Behavior"; overflow "Overflow Behavior"; add_latency "Add Latency"; mult_latency "Mult Latency"; bram_latency "BRAM Latency"
      mask init: same as fft_test/fft/fft_biplex0/biplex_core/fft_stage_1
      settings: AttributesFormatString=FFTSize=4, FFTStage=2, BitWidth=8
      mask StyleString: edit,edit,edit,edit,edit,edit,popup(Truncate|Round  (unbiased: +/- Inf)|Round  (unbiased: Even Values)),popup(Wrap|Saturate|Error),edit,edit,edit
  fft_stage_3 : Subsystem  AncestorBlock=casper_library/FFTs/fft_stage_n  mask(fft_stage_n){FFTSize=4, FFTStage=3, BitWidth=8, use_bram=0, CoeffBram=0, MaxCoeffNum=11, quantization=Round  (unbiased: +/- Inf), overflow=Saturate, add_latency=2, mult_latency=3, bram_latency=1}
      mask prompts: FFTSize "Size of FFT: (2^? pnts)"; FFTStage "Stage of FFT:"; BitWidth "Output Bitwidth:"; use_bram "Implement Delays in BRAM:"; CoeffBram "Store Coefficients in BRAM:"; MaxCoeffNum "Maximum Coefficient Depth: (2^?)"; quantization "Quantization Behavior"; overflow "Overflow Behavior"; add_latency "Add Latency"; mult_latency "Mult Latency"; bram_latency "BRAM Latency"
      mask init: same as fft_test/fft/fft_biplex0/biplex_core/fft_stage_1
      settings: AttributesFormatString=FFTSize=4, FFTStage=3, BitWidth=8
      mask StyleString: edit,edit,edit,edit,edit,edit,popup(Truncate|Round  (unbiased: +/- Inf)|Round  (unbiased: Even Values)),popup(Wrap|Saturate|Error),edit,edit,edit
  fft_stage_4 : Subsystem  AncestorBlock=casper_library/FFTs/fft_stage_n  mask(fft_stage_n){FFTSize=4, FFTStage=4, BitWidth=8, use_bram=0, CoeffBram=0, MaxCoeffNum=11, quantization=Round  (unbiased: +/- Inf), overflow=Saturate, add_latency=2, mult_latency=3, bram_latency=1}
      mask prompts: FFTSize "Size of FFT: (2^? pnts)"; FFTStage "Stage of FFT:"; BitWidth "Output Bitwidth:"; use_bram "Implement Delays in BRAM:"; CoeffBram "Store Coefficients in BRAM:"; MaxCoeffNum "Maximum Coefficient Depth: (2^?)"; quantization "Quantization Behavior"; overflow "Overflow Behavior"; add_latency "Add Latency"; mult_latency "Mult Latency"; bram_latency "BRAM Latency"
      mask init: same as fft_test/fft/fft_biplex0/biplex_core/fft_stage_1
      settings: AttributesFormatString=FFTSize=4, FFTStage=4, BitWidth=8
      mask StyleString: edit,edit,edit,edit,edit,edit,popup(Truncate|Round  (unbiased: +/- Inf)|Round  (unbiased: Even Values)),popup(Wrap|Saturate|Error),edit,edit,edit
  out1 : Outport  OutDataType=sfix(16)  OutScaling=2^0
  out2 : Outport  Port=2  OutDataType=sfix(16)  OutScaling=2^0
  of : Outport  Port=3  OutDataType=sfix(16)  OutScaling=2^0
  sync_out : Outport  Port=4  OutDataType=sfix(16)  OutScaling=2^0
  wires:
  fft_stage_1/1(out1) -> fft_stage_2/1(in1)
  fft_stage_1/2(out2) -> fft_stage_2/2(in2)
  fft_stage_1/3(of) -> fft_stage_2/3(of_in)
  fft_stage_1/4(sync_out) -> fft_stage_2/4(sync)
  shift/1 -> fft_stage_2/5(shift), fft_stage_3/5(shift), fft_stage_4/5(shift), fft_stage_1/4(shift)
  fft_stage_2/1(out1) -> fft_stage_3/1(in1)
  fft_stage_2/2(out2) -> fft_stage_3/2(in2)
  fft_stage_2/3(of) -> fft_stage_3/3(of_in)
  fft_stage_2/4(sync_out) -> fft_stage_3/4(sync)
  fft_stage_3/1(out1) -> fft_stage_4/1(in1)
  fft_stage_3/2(out2) -> fft_stage_4/2(in2)
  fft_stage_3/3(of) -> fft_stage_4/3(of_in)
  fft_stage_3/4(sync_out) -> fft_stage_4/4(sync)
  pol1/1 -> fft_stage_1/1(in1)
  pol2/1 -> fft_stage_1/2(in2)
  sync/1 -> fft_stage_1/3(sync)
  fft_stage_4/1(out1) -> out1/1
  fft_stage_4/2(out2) -> out2/1
  fft_stage_4/3(of) -> of/1
  fft_stage_4/4(sync_out) -> sync_out/1

== system fft_test/fft/fft_biplex0/biplex_cplx_unscrambler ==
  even : Inport  OutDataType=sfix(16)  OutScaling=2^0
  odd : Inport  Port=2  OutDataType=sfix(16)  OutScaling=2^0
  sync : Inport  Port=3  OutDataType=sfix(16)  OutScaling=2^0
  Constant : xbsIndex_r4/Constant  arith_type=Boolean  const=1  n_bits=1  bin_pt=0  explicit_period=on  period=1  equ=P=C  opselect=C  inp2=PCIN>>17  opr=+  inp1=P  carry=CIN  dbl_ovrd=off  block_type=constant
      settings: block_version=9.1.01
  Constant1 : xbsIndex_r4/Constant  arith_type=Unsigned  const=2^(FFTSize-1)  n_bits=FFTSize  bin_pt=0  explicit_period=on  period=1  equ=P=C  opselect=C  inp2=PCIN>>17  opr=+  inp1=P  carry=CIN  dbl_ovrd=off  block_type=constant
      settings: block_version=9.1.01
  Constant2 : xbsIndex_r4/Constant  arith_type=Unsigned  const=2^(FFTSize-1)  n_bits=FFTSize  bin_pt=0  explicit_period=on  period=1  equ=P=C  opselect=C  inp2=PCIN>>17  opr=+  inp1=P  carry=CIN  dbl_ovrd=off  block_type=constant
      settings: block_version=9.1.01
  Convert : xbsIndex_r4/Convert  arith_type=Unsigned  n_bits=1  bin_pt=0  quantization=Truncate  overflow=Wrap  latency=0  dbl_ovrd=off  pipeline=off  block_type=convert
      settings: xl_area=[0, 0, 0, 0, 0, 0, 0]
  Convert1 : xbsIndex_r4/Convert  arith_type=Unsigned  n_bits=1  bin_pt=0  quantization=Truncate  overflow=Wrap  latency=0  dbl_ovrd=off  pipeline=off  block_type=convert
      settings: xl_area=[0, 0, 0, 0, 0, 0, 0]
  Counter : xbsIndex_r4/Counter  cnt_type=Free Running  cnt_to=Inf  operation=Up  start_count=0  cnt_by_val=1  arith_type=Unsigned  n_bits=FFTSize  bin_pt=0  load_pin=off  rst=on  en=off  explicit_period=off  period=1  dbl_ovrd=off  use_behavioral_HDL=off  use_rpm=on  block_type=counter
      settings: xl_area=[0, 0, 0, 0, 0, 0, 0]  block_version=9.1.01
  Counter1 : xbsIndex_r4/Counter  cnt_type=Free Running  cnt_to=Inf  operation=Up  start_count=0  cnt_by_val=1  arith_type=Unsigned  n_bits=FFTSize  bin_pt=0  load_pin=off  rst=on  en=off  explicit_period=off  period=1  dbl_ovrd=off  use_behavioral_HDL=off  use_rpm=on  block_type=counter
      settings: xl_area=[0, 0, 0, 0, 0, 0, 0]  block_version=9.1.01
  Relational : xbsIndex_r4/Relational  mode=a<=b  en=off  latency=0  dbl_ovrd=off  block_type=relational
      settings: xl_area=[0, 0, 0, 0, 0, 0, 0]  block_version=9.1.01
  Relational1 : xbsIndex_r4/Relational  mode=a<=b  en=off  latency=0  dbl_ovrd=off  block_type=relational
      settings: xl_area=[0, 0, 0, 0, 0, 0, 0]  block_version=9.1.01
  barrel_switcher : casper_library/Reorder/barrel_switcher  SystemSampleTime=-1  n_inputs=1
      settings: AttributesFormatString=n_inputs=1
  barrel_switcher1 : casper_library/Reorder/barrel_switcher  SystemSampleTime=-1  n_inputs=1
      settings: AttributesFormatString=n_inputs=1
  reorder : Subsystem  AncestorBlock=casper_library/Reorder/reorder  mask(reorder){map=[0 4 2 6 1 5 3 7 8 12 10 14 9 13 11 15], n_inputs=1, bram_latency=1, map_latency=0, double_buffer=0}
      mask prompts: map "Output Order:"; n_inputs "Number of inputs"; bram_latency "BRAM Latency"; map_latency "Map Latency"; double_buffer "Double Buffer"
      mask init:
      | reorder_init(gcb, ...
      |     'map', map, ...
      |     'n_inputs', n_inputs, ...
      |     'bram_latency', bram_latency, ...
      |     'map_latency', map_latency, ...
      |     'double_buffer', double_buffer);
      settings: AttributesFormatString=order=2
  reorder1 : Subsystem  AncestorBlock=casper_library/Reorder/reorder  mask(reorder){map=[8 12 10 14 9 13 11 15 0 4 2 6 1 5 3 7], n_inputs=1, bram_latency=1, map_latency=0, double_buffer=0}
      mask prompts: map "Output Order:"; n_inputs "Number of inputs"; bram_latency "BRAM Latency"; map_latency "Map Latency"; double_buffer "Double Buffer"
      mask init:
      | reorder_init(gcb, ...
      |     'map', map, ...
      |     'n_inputs', n_inputs, ...
      |     'bram_latency', bram_latency, ...
      |     'map_latency', map_latency, ...
      |     'double_buffer', double_buffer);
      settings: AttributesFormatString=order=2
  pol1 : Outport  OutDataType=sfix(16)  OutScaling=2^0
  pol2 : Outport  Port=2  OutDataType=sfix(16)  OutScaling=2^0
  sync_out : Outport  Port=3  OutDataType=sfix(16)  OutScaling=2^0
  wires:
  Convert/1 -> barrel_switcher/1
  Convert1/1 -> barrel_switcher1/1
  Relational1/1 -> Convert1/1
  Relational/1 -> Convert/1
  Constant2/1 -> Relational1/1
  Counter1/1 -> Relational1/2
  Counter/1 -> Relational/2
  Constant1/1 -> Relational/1
  Constant/1 -> reorder1/2(en), reorder/2(en)
  sync/1 -> Counter/1, barrel_switcher/2
  barrel_switcher1/3 -> pol2/1
  barrel_switcher1/2 -> pol1/1
  barrel_switcher1/1 -> sync_out/1
  odd/1 -> barrel_switcher/4
  even/1 -> barrel_switcher/3
  reorder1/3(dout0) -> barrel_switcher1/4
  reorder/3(dout0) -> barrel_switcher1/3
  reorder/1(sync_out) -> Counter1/1, barrel_switcher1/2
  barrel_switcher/3 -> reorder1/3(din0)
  barrel_switcher/2 -> reorder/3(din0)
  barrel_switcher/1 -> reorder1/1(sync), reorder/1(sync)

== system fft_test/fft/fft_biplex1/biplex_core ==
  pol1 : Inport  OutDataType=sfix(16)  OutScaling=2^0
  pol2 : Inport  Port=2  OutDataType=sfix(16)  OutScaling=2^0
  sync : Inport  Port=3  OutDataType=sfix(16)  OutScaling=2^0
  shift : Inport  Port=4  OutDataType=sfix(16)  OutScaling=2^0
  fft_stage_1 : Subsystem  mask(fft_stage_n){FFTSize=4, FFTStage=1, BitWidth=8, use_bram=0, CoeffBram=0, MaxCoeffNum=11, quantization=Round  (unbiased: +/- Inf), overflow=Saturate, add_latency=2, mult_latency=3, bram_latency=1}
      mask prompts: FFTSize "Size of FFT: (2^? pnts)"; FFTStage "Stage of FFT:"; BitWidth "Output Bitwidth:"; use_bram "Implement Delays in BRAM:"; CoeffBram "Store Coefficients in BRAM:"; MaxCoeffNum "Maximum Coefficient Depth: (2^?)"; quantization "Quantization Behavior"; overflow "Overflow Behavior"; add_latency "Add Latency"; mult_latency "Mult Latency"; bram_latency "BRAM Latency"
      mask init: same as fft_test/fft/fft_biplex0/biplex_core/fft_stage_1
      settings: AttributesFormatString=FFTSize=4, FFTStage=1, BitWidth=8
      mask StyleString: edit,edit,edit,edit,edit,edit,popup(Truncate|Round  (unbiased: +/- Inf)|Round  (unbiased: Even Values)),popup(Wrap|Saturate|Error),edit,edit,edit
  fft_stage_2 : Subsystem  AncestorBlock=casper_library/FFTs/fft_stage_n  mask(fft_stage_n){FFTSize=4, FFTStage=2, BitWidth=8, use_bram=0, CoeffBram=0, MaxCoeffNum=11, quantization=Round  (unbiased: +/- Inf), overflow=Saturate, add_latency=2, mult_latency=3, bram_latency=1}
      mask prompts: FFTSize "Size of FFT: (2^? pnts)"; FFTStage "Stage of FFT:"; BitWidth "Output Bitwidth:"; use_bram "Implement Delays in BRAM:"; CoeffBram "Store Coefficients in BRAM:"; MaxCoeffNum "Maximum Coefficient Depth: (2^?)"; quantization "Quantization Behavior"; overflow "Overflow Behavior"; add_latency "Add Latency"; mult_latency "Mult Latency"; bram_latency "BRAM Latency"
      mask init: same as fft_test/fft/fft_biplex0/biplex_core/fft_stage_1
      settings: AttributesFormatString=FFTSize=4, FFTStage=2, BitWidth=8
      mask StyleString: edit,edit,edit,edit,edit,edit,popup(Truncate|Round  (unbiased: +/- Inf)|Round  (unbiased: Even Values)),popup(Wrap|Saturate|Error),edit,edit,edit
  fft_stage_3 : Subsystem  AncestorBlock=casper_library/FFTs/fft_stage_n  mask(fft_stage_n){FFTSize=4, FFTStage=3, BitWidth=8, use_bram=0, CoeffBram=0, MaxCoeffNum=11, quantization=Round  (unbiased: +/- Inf), overflow=Saturate, add_latency=2, mult_latency=3, bram_latency=1}
      mask prompts: FFTSize "Size of FFT: (2^? pnts)"; FFTStage "Stage of FFT:"; BitWidth "Output Bitwidth:"; use_bram "Implement Delays in BRAM:"; CoeffBram "Store Coefficients in BRAM:"; MaxCoeffNum "Maximum Coefficient Depth: (2^?)"; quantization "Quantization Behavior"; overflow "Overflow Behavior"; add_latency "Add Latency"; mult_latency "Mult Latency"; bram_latency "BRAM Latency"
      mask init: same as fft_test/fft/fft_biplex0/biplex_core/fft_stage_1
      settings: AttributesFormatString=FFTSize=4, FFTStage=3, BitWidth=8
      mask StyleString: edit,edit,edit,edit,edit,edit,popup(Truncate|Round  (unbiased: +/- Inf)|Round  (unbiased: Even Values)),popup(Wrap|Saturate|Error),edit,edit,edit
  fft_stage_4 : Subsystem  AncestorBlock=casper_library/FFTs/fft_stage_n  mask(fft_stage_n){FFTSize=4, FFTStage=4, BitWidth=8, use_bram=0, CoeffBram=0, MaxCoeffNum=11, quantization=Round  (unbiased: +/- Inf), overflow=Saturate, add_latency=2, mult_latency=3, bram_latency=1}
      mask prompts: FFTSize "Size of FFT: (2^? pnts)"; FFTStage "Stage of FFT:"; BitWidth "Output Bitwidth:"; use_bram "Implement Delays in BRAM:"; CoeffBram "Store Coefficients in BRAM:"; MaxCoeffNum "Maximum Coefficient Depth: (2^?)"; quantization "Quantization Behavior"; overflow "Overflow Behavior"; add_latency "Add Latency"; mult_latency "Mult Latency"; bram_latency "BRAM Latency"
      mask init: same as fft_test/fft/fft_biplex0/biplex_core/fft_stage_1
      settings: AttributesFormatString=FFTSize=4, FFTStage=4, BitWidth=8
      mask StyleString: edit,edit,edit,edit,edit,edit,popup(Truncate|Round  (unbiased: +/- Inf)|Round  (unbiased: Even Values)),popup(Wrap|Saturate|Error),edit,edit,edit
  out1 : Outport  OutDataType=sfix(16)  OutScaling=2^0
  out2 : Outport  Port=2  OutDataType=sfix(16)  OutScaling=2^0
  of : Outport  Port=3  OutDataType=sfix(16)  OutScaling=2^0
  sync_out : Outport  Port=4  OutDataType=sfix(16)  OutScaling=2^0
  wires:
  fft_stage_1/1(out1) -> fft_stage_2/1(in1)
  fft_stage_1/2(out2) -> fft_stage_2/2(in2)
  fft_stage_1/3(of) -> fft_stage_2/3(of_in)
  fft_stage_1/4(sync_out) -> fft_stage_2/4(sync)
  shift/1 -> fft_stage_2/5(shift), fft_stage_3/5(shift), fft_stage_4/5(shift), fft_stage_1/4(shift)
  fft_stage_2/1(out1) -> fft_stage_3/1(in1)
  fft_stage_2/2(out2) -> fft_stage_3/2(in2)
  fft_stage_2/3(of) -> fft_stage_3/3(of_in)
  fft_stage_2/4(sync_out) -> fft_stage_3/4(sync)
  fft_stage_3/1(out1) -> fft_stage_4/1(in1)
  fft_stage_3/2(out2) -> fft_stage_4/2(in2)
  fft_stage_3/3(of) -> fft_stage_4/3(of_in)
  fft_stage_3/4(sync_out) -> fft_stage_4/4(sync)
  pol1/1 -> fft_stage_1/1(in1)
  pol2/1 -> fft_stage_1/2(in2)
  sync/1 -> fft_stage_1/3(sync)
  fft_stage_4/1(out1) -> out1/1
  fft_stage_4/2(out2) -> out2/1
  fft_stage_4/3(of) -> of/1
  fft_stage_4/4(sync_out) -> sync_out/1

== system fft_test/fft/fft_biplex1/biplex_cplx_unscrambler ==
  even : Inport  OutDataType=sfix(16)  OutScaling=2^0
  odd : Inport  Port=2  OutDataType=sfix(16)  OutScaling=2^0
  sync : Inport  Port=3  OutDataType=sfix(16)  OutScaling=2^0
  Constant : xbsIndex_r4/Constant  arith_type=Boolean  const=1  n_bits=1  bin_pt=0  explicit_period=on  period=1  equ=P=C  opselect=C  inp2=PCIN>>17  opr=+  inp1=P  carry=CIN  dbl_ovrd=off  block_type=constant
      settings: block_version=9.1.01
  Constant1 : xbsIndex_r4/Constant  arith_type=Unsigned  const=2^(FFTSize-1)  n_bits=FFTSize  bin_pt=0  explicit_period=on  period=1  equ=P=C  opselect=C  inp2=PCIN>>17  opr=+  inp1=P  carry=CIN  dbl_ovrd=off  block_type=constant
      settings: block_version=9.1.01
  Constant2 : xbsIndex_r4/Constant  arith_type=Unsigned  const=2^(FFTSize-1)  n_bits=FFTSize  bin_pt=0  explicit_period=on  period=1  equ=P=C  opselect=C  inp2=PCIN>>17  opr=+  inp1=P  carry=CIN  dbl_ovrd=off  block_type=constant
      settings: block_version=9.1.01
  Convert : xbsIndex_r4/Convert  arith_type=Unsigned  n_bits=1  bin_pt=0  quantization=Truncate  overflow=Wrap  latency=0  dbl_ovrd=off  pipeline=off  block_type=convert
      settings: xl_area=[0, 0, 0, 0, 0, 0, 0]
  Convert1 : xbsIndex_r4/Convert  arith_type=Unsigned  n_bits=1  bin_pt=0  quantization=Truncate  overflow=Wrap  latency=0  dbl_ovrd=off  pipeline=off  block_type=convert
      settings: xl_area=[0, 0, 0, 0, 0, 0, 0]
  Counter : xbsIndex_r4/Counter  cnt_type=Free Running  cnt_to=Inf  operation=Up  start_count=0  cnt_by_val=1  arith_type=Unsigned  n_bits=FFTSize  bin_pt=0  load_pin=off  rst=on  en=off  explicit_period=off  period=1  dbl_ovrd=off  use_behavioral_HDL=off  use_rpm=on  block_type=counter
      settings: xl_area=[0, 0, 0, 0, 0, 0, 0]  block_version=9.1.01
  Counter1 : xbsIndex_r4/Counter  cnt_type=Free Running  cnt_to=Inf  operation=Up  start_count=0  cnt_by_val=1  arith_type=Unsigned  n_bits=FFTSize  bin_pt=0  load_pin=off  rst=on  en=off  explicit_period=off  period=1  dbl_ovrd=off  use_behavioral_HDL=off  use_rpm=on  block_type=counter
      settings: xl_area=[0, 0, 0, 0, 0, 0, 0]  block_version=9.1.01
  Relational : xbsIndex_r4/Relational  mode=a<=b  en=off  latency=0  dbl_ovrd=off  block_type=relational
      settings: xl_area=[0, 0, 0, 0, 0, 0, 0]  block_version=9.1.01
  Relational1 : xbsIndex_r4/Relational  mode=a<=b  en=off  latency=0  dbl_ovrd=off  block_type=relational
      settings: xl_area=[0, 0, 0, 0, 0, 0, 0]  block_version=9.1.01
  barrel_switcher : casper_library/Reorder/barrel_switcher  SystemSampleTime=-1  n_inputs=1
      settings: AttributesFormatString=n_inputs=1
  barrel_switcher1 : casper_library/Reorder/barrel_switcher  SystemSampleTime=-1  n_inputs=1
      settings: AttributesFormatString=n_inputs=1
  reorder : Subsystem  AncestorBlock=casper_library/Reorder/reorder  mask(reorder){map=[0 4 2 6 1 5 3 7 8 12 10 14 9 13 11 15], n_inputs=1, bram_latency=1, map_latency=0, double_buffer=0}
      mask prompts: map "Output Order:"; n_inputs "Number of inputs"; bram_latency "BRAM Latency"; map_latency "Map Latency"; double_buffer "Double Buffer"
      mask init:
      | reorder_init(gcb, ...
      |     'map', map, ...
      |     'n_inputs', n_inputs, ...
      |     'bram_latency', bram_latency, ...
      |     'map_latency', map_latency, ...
      |     'double_buffer', double_buffer);
      settings: AttributesFormatString=order=2
  reorder1 : Subsystem  AncestorBlock=casper_library/Reorder/reorder  mask(reorder){map=[8 12 10 14 9 13 11 15 0 4 2 6 1 5 3 7], n_inputs=1, bram_latency=1, map_latency=0, double_buffer=0}
      mask prompts: map "Output Order:"; n_inputs "Number of inputs"; bram_latency "BRAM Latency"; map_latency "Map Latency"; double_buffer "Double Buffer"
      mask init:
      | reorder_init(gcb, ...
      |     'map', map, ...
      |     'n_inputs', n_inputs, ...
      |     'bram_latency', bram_latency, ...
      |     'map_latency', map_latency, ...
      |     'double_buffer', double_buffer);
      settings: AttributesFormatString=order=2
  pol1 : Outport  OutDataType=sfix(16)  OutScaling=2^0
  pol2 : Outport  Port=2  OutDataType=sfix(16)  OutScaling=2^0
  sync_out : Outport  Port=3  OutDataType=sfix(16)  OutScaling=2^0
  wires:
  Convert/1 -> barrel_switcher/1
  Convert1/1 -> barrel_switcher1/1
  Relational1/1 -> Convert1/1
  Relational/1 -> Convert/1
  Constant2/1 -> Relational1/1
  Counter1/1 -> Relational1/2
  Counter/1 -> Relational/2
  Constant1/1 -> Relational/1
  Constant/1 -> reorder1/2(en), reorder/2(en)
  sync/1 -> Counter/1, barrel_switcher/2
  barrel_switcher1/3 -> pol2/1
  barrel_switcher1/2 -> pol1/1
  barrel_switcher1/1 -> sync_out/1
  odd/1 -> barrel_switcher/4
  even/1 -> barrel_switcher/3
  reorder1/3(dout0) -> barrel_switcher1/4
  reorder/3(dout0) -> barrel_switcher1/3
  reorder/1(sync_out) -> Counter1/1, barrel_switcher1/2
  barrel_switcher/3 -> reorder1/3(din0)
  barrel_switcher/2 -> reorder/3(din0)
  barrel_switcher/1 -> reorder1/1(sync), reorder/1(sync)
